simulink model "pp_control_sim"  (R2025b)
settings: Solver=VariableStepAuto  StartTime=0.0  StopTime=0.5  RelTol=1e-3
values from neighbouring files (symbols this model uses):
  A = [-Ra/La, -Kb/La,  0 ... (first row only)    [pp_control_src.m]
  B = [1/La ... (first row only)    [pp_control_src.m]
  C = [0, 0, 1]    [pp_control_src.m]
  K = place(A, B, P)    [pp_control_src.m]
  K_dc = 1 / dcgain(sys_cl_sin_ajuste)    [pp_control_src.m]
settings Model: Creator=maxvega  LastModifiedBy=maxvega

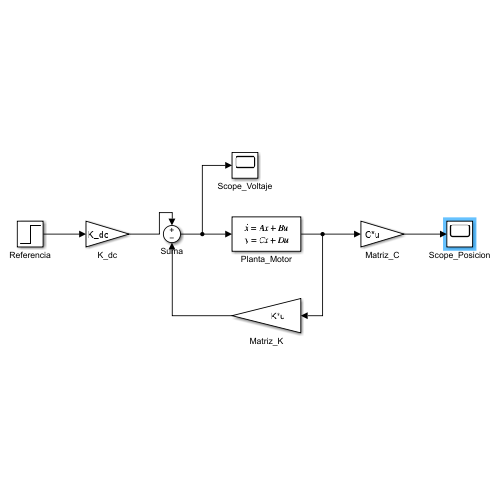
[thumbnail: Simulink's stored preview of the top-level diagram]
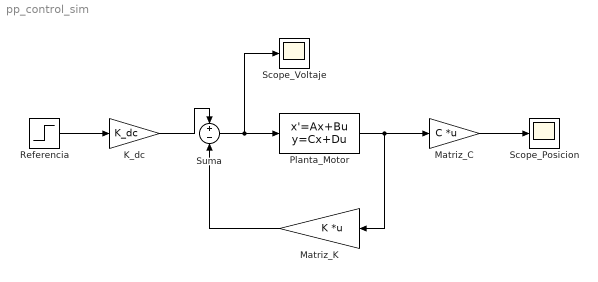
== system pp_control_sim ==
  K_dc : Gain  Gain=K_dc
  Matriz_C : Gain  Gain=C  Multiplication=Matrix(K*u)
  Matriz_K : Gain  Gain=K  Multiplication=Matrix(K*u)
  Planta_Motor : StateSpace  A=A  B=B  C=eye(3)  D=zeros(3,1)  InitialCondition=0
  Referencia : Step  Time=0  SampleTime=0
  Scope_Posicion : Scope
      settings: ActiveDisplayYMinimum=-0.17144977556713373  ActiveDisplayYMaximum=1.5430479801042039
  Scope_Voltaje : Scope
  Suma : Sum  Inputs=+-
  wires:
  Referencia/1 -> K_dc/1
  K_dc/1 -> Suma/1
  Suma/1 -> Planta_Motor/1, Scope_Voltaje/1
  Planta_Motor/1 -> Matriz_C/1, Matriz_K/1
  Matriz_C/1 -> Scope_Posicion/1
  Matriz_K/1 -> Suma/2
